simulink model "part4_Final_Project"  (R2016b)
settings: Solver=FixedStepDiscrete  StartTime=0.0  StopTime=inf  FixedStep=.03  RelTol=1e-3  EnableMultiTasking=on
undefined symbols (not defined in the file or in its folder): Klqr
libraries: arduinolib x2, simulink x1
settings Model: SimulationMode=external  ExtModeTrigDuration=2  Creator=008528533  LastModifiedBy=Mac
settings DataIOCC: LimitDataPoints=on  SaveFormat=Array
settings OptimizationCC: LifeSpan=1
settings DebuggingCC: UnderspecifiedInitializationDetection=Classic  MergeDetectMultiDrivingBlocksExec=none  SFUnexpectedBacktrackingDiag=warning  SFNoUnconditionalDefaultTransitionDiag=warning  SFExecutionAtInitializationDiag=none
settings HardwareCC: ProdBitPerInt=16  ProdBitPerPointer=8  ProdBitPerSizeT=16  ProdBitPerPtrDiffT=16  ProdLargestAtomicFloat=None  ProdWordSize=8  ProdHWDeviceType=Atmel->AVR
settings ModelReferenceCC: PropagateSignalLabelsOutOfModel=off
settings RTWCC: SystemTargetFile=realtime.tlc  GenerateMakefile=off  TemplateMakefile=realtime.tmf  Description=Run on Target Hardware  RTWVerbose=off
settings STFCustomTargetCC: TargetLibSuffix=.a  GenerateSampleERTMain=on  ERTCustomFileBanners=on  SupportNonInlinedSFcns=off  RemoveResetFunc=on  SupportVariableSizeSignals=on  MATLABClassNameForMDSCustomization=Simulink.SoftwareTarget.ERTCustomization  GRTInterface=off  SystemTargetFile=realtime.tlc
settings ERTTargetCC: GenerateSampleERTMain=on  ParMdlRefBuildCompliant=off  CompOptLevelCompliant=off  ConcurrentExecutionCompliant=off  CombineOutputUpdateFcns=off  ERTFirstTimeCompliant=off  SupportContinuousTime=on  SupportVariableSizeSignals=on  ModelStepFunctionPrototypeControlCompliant=off  CPPClassGenCompliant=off  UseToolchainInfoCompliant=off  ExtMode=on  ExtModeTransport=3  ExtModeMexFile=ext_serial_win32_comm_rtt  ExtModeMexArgs=0 8 115200 30  ERTSrcFileBannerTemplate=realtime_code_template.cgt  ERTHdrFileBannerTemplate=realtime_code_template.cgt  ERTDataSrcFileTemplate=realtime_code_template.cgt  ERTDataHdrFileTemplate=realtime_code_template.cgt  ERTCustomFileTemplate=realtime_file_process.tlc  ConvertIfToSwitch=off  SuppressUnreachableDefaultCases=off
settings ConfigComp: CovMetricSettings=dw  CovHtmlReporting=on  CovSaveCumulativeToWorkspaceVar=on  CovSaveSingleToWorkspaceVar=on  CovExternalEMLEnable=off

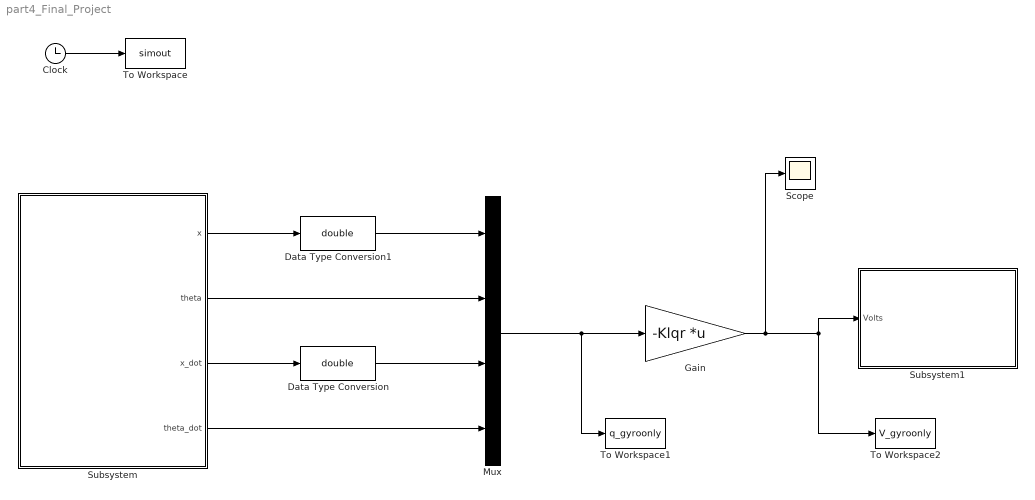
== system part4_Final_Project ==
  Clock : Clock
  Data Type Conversion : DataTypeConversion  OutDataTypeStr=double
  Data Type Conversion1 : DataTypeConversion  OutDataTypeStr=double
  Gain : Gain  Gain=-Klqr  Multiplication=Matrix(K*u)
  Mux : Mux
  Scope : Scope
  Subsystem : Subsystem
  Subsystem1 : Subsystem
  To Workspace : ToWorkspace  VariableName=simout  SaveFormat=Timeseries  SampleTime=-1
  To Workspace1 : ToWorkspace  VariableName=q_gyroonly  SampleTime=-1
  To Workspace2 : ToWorkspace  VariableName=V_gyroonly  SampleTime=-1
  wires:
  Clock/1 -> To Workspace/1
  Subsystem/1(x) -> Data Type Conversion1/1
  Data Type Conversion1/1 -> Mux/1
  Subsystem/2("theta ") -> Mux/2
  Subsystem/3(x_dot) -> Data Type Conversion/1
  Data Type Conversion/1 -> Mux/3
  Subsystem/4("theta_dot ") -> Mux/4
  Mux/1 -> To Workspace1/1, Gain/1
  Gain/1 -> Scope/1, To Workspace2/1, Subsystem1/1(Volts)

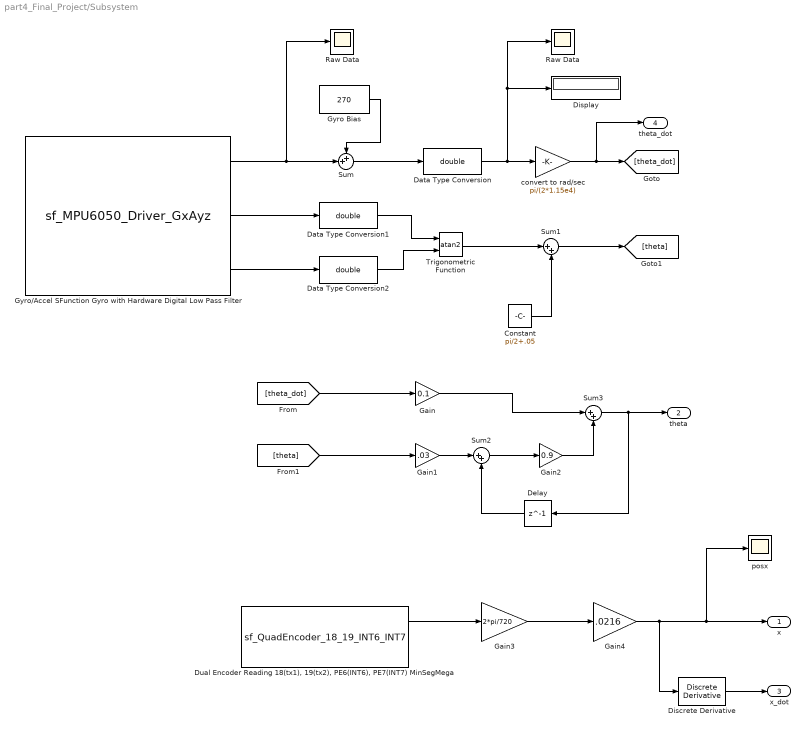
== system part4_Final_Project/Subsystem ==
  Constant : Constant  Value=pi/2+.05
  Data Type Conversion : DataTypeConversion  OutDataTypeStr=double
  Data Type Conversion1 : DataTypeConversion  OutDataTypeStr=double
  Data Type Conversion2 : DataTypeConversion  OutDataTypeStr=double
  Delay : Delay  DelayLength=1
  Discrete Derivative : simulink/Discrete/Discrete Derivative  gainval=1.0  ICPrevScaledInput=0.0  InputProcessing=Inherited  OutMin=[]  OutMax=[]  OutDataType=fixdt(1, 16)  OutScaling=2^-10  DoSatur=off
  Display : Display
  "Dual Encoder Reading 18(tx1), 19(tx2), PE6(INT6), PE7(INT7) MinSegMega " : S-Function  InitFcn=try, set_param(gcb,'FunctionName','sf_QuadEncoder_18_19_INT6_INT7'), end  FunctionName=sf_QuadEncoder_18_19_INT6_INT7  Parameters=uint8([0 1]),uint8([18 6]),uint8([19 7])  SFunctionModules=sf_QuadEncoder_18_19_INT6_INT7_wrapper  SFunctionDeploymentMode=off  EnableBusSupport=off  mask(S-Function Builder){}
      mask init:
      | val = [[.9  0.75 0.75 1 1 .9 .9 1]',[1 1 0.75 0.75 .9 .9 1 .9]'];try , sys = get_param(gcb,'SfunBuilderFcnName');if isempty(sys), sys = get_param(gcb,'FunctionName'); end,catch, sys = get_param(gcb,'FunctionName'); end
      settings: CopyFcn=set_param(gcbh,'LinkStatus','none')  PreSaveFcn=try, set_param(gcb,'FunctionName','sf_QuadEncoder_18_19_INT6_INT7'), end  OpenFcn=sfunctionwizard(gcbh)
      mask Display: plot(val(:,1),val(:,2)),disp(sys), port_label('output',1,'pos1'), port_label('output',2,'pos2')
  Gain : Gain  Gain=0.1
  Gain1 : Gain  Gain=.03
  Gain2 : Gain  Gain=0.9
  Gain3 : Gain  Gain=2*pi/720
  Gain4 : Gain  Gain=.0216
  Gyro Bias : Constant  Value=270
  Gyro/Accel SFunction Gyro with Hardware Digital Low Pass Filter : S-Function  InitFcn=try, set_param(gcb,'FunctionName','sf_MPU6050_Driver_GxAyz'), end  FunctionName=sf_MPU6050_Driver_GxAyz  SFunctionModules=sf_MPU6050_Driver_GxAyz_wrapper  SFunctionDeploymentMode=off  EnableBusSupport=off  mask(S-Function Builder){}
      mask help: Simulink:masks:SFunctionBuilder_MD
      mask init: same as part4_Final_Project/Subsystem/Dual Encoder Reading 18(tx1), 19(tx2), PE6(INT6), PE7(INT7) MinSegMega 
      settings: CopyFcn=set_param(gcbh,'LinkStatus','none')  PreSaveFcn=try, set_param(gcb,'FunctionName','sf_MPU6050_Driver_GxAyz'), end  OpenFcn=sfunctionwizard(gcbh)
      mask Display: plot(val(:,1),val(:,2)),disp(sys), port_label('output',1,'x_vel'), port_label('output',2,'y_acc'), port_label('output',3,'z_acc')
  Raw Data : Scope
  "Raw Data " : Scope
  Sum : Sum  Inputs=++|
  Sum1 : Sum  Inputs=|++
  Sum2 : Sum  Inputs=|++
  Sum3 : Sum  Inputs=|++
  Trigonometric Function : Trigonometry  Operator=atan2
  convert to rad/sec : Gain  Gain=pi/(2*1.15e4)
  posx : Scope
  x : Outport
  "theta " : Outport  Port=2
  x_dot : Outport  Port=3
  "theta_dot " : Outport  Port=4
  wires:
  Gyro Bias/1 -> Sum/1
  Sum/1 -> Data Type Conversion/1
  Data Type Conversion/1 -> Raw Data/1, Display/1, convert to rad/sec/1
  convert to rad/sec/1 -> "theta_dot "/1, [theta_dot]
  Gyro/Accel SFunction Gyro with Hardware Digital Low Pass Filter/1 -> "Raw Data "/1, Sum/2
  Gyro/Accel SFunction Gyro with Hardware Digital Low Pass Filter/3 -> Data Type Conversion2/1
  Gyro/Accel SFunction Gyro with Hardware Digital Low Pass Filter/2 -> Data Type Conversion1/1
  Data Type Conversion1/1 -> Trigonometric Function/1
  Trigonometric Function/1 -> Sum1/1
  Data Type Conversion2/1 -> Trigonometric Function/2
  [theta_dot] -> Gain/1
  Constant/1 -> Sum1/2
  Sum1/1 -> [theta]
  [theta] -> Gain1/1
  Sum3/1 -> "theta "/1, Delay/1
  Delay/1 -> Sum2/2
  Sum2/1 -> Gain2/1
  Gain1/1 -> Sum2/1
  Gain/1 -> Sum3/1
  Gain2/1 -> Sum3/2
  Gain3/1 -> Gain4/1
  "Dual Encoder Reading 18(tx1), 19(tx2), PE6(INT6), PE7(INT7) MinSegMega "/1 -> Gain3/1
  Gain4/1 -> posx/1, x/1, Discrete Derivative/1
  Discrete Derivative/1 -> x_dot/1

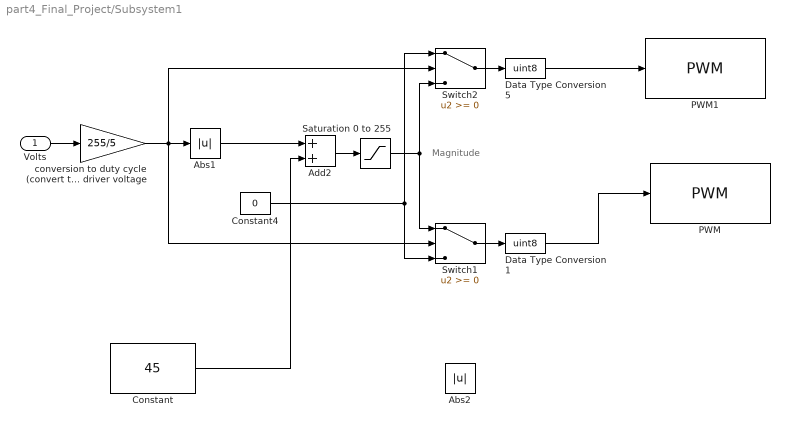
== system part4_Final_Project/Subsystem1 ==
  note: Magnitude
  Volts : Inport
  Abs1 : Abs
  Abs2 : Abs
  Add2 : Sum
  Constant : Constant  Value=45
  Constant4 : Constant  Value=0
  Data Type Conversion1 : DataTypeConversion  OutDataTypeStr=uint8
  Data Type Conversion5 : DataTypeConversion  OutDataTypeStr=uint8
  PWM : arduinolib/PWM  pinNumber=45  blockPlatform=arduino
  PWM1 : arduinolib/PWM  pinNumber=44  blockPlatform=arduino
  Saturation 0 to 255 : Saturate  UpperLimit=255  LowerLimit=0
  Switch1 : Switch
  Switch2 : Switch
  conversion to duty cycle (convert to int) denominator is motor driver voltage : Gain  Gain=255/5  OutDataTypeStr=int16
  wires:
  Volts/1 -> conversion to duty cycle (convert to int) denominator is motor driver voltage/1
  conversion to duty cycle (convert to int) denominator is motor driver voltage/1 -> Abs1/1, Switch2/2, Switch1/2
  Switch2/1 -> Data Type Conversion5/1
  Constant4/1 -> Switch1/3, Switch2/1
  Switch1/1 -> Data Type Conversion1/1
  Data Type Conversion1/1 -> PWM/1
  Data Type Conversion5/1 -> PWM1/1
  Constant/1 -> Add2/2
  Add2/1 -> Saturation 0 to 255/1
  Abs1/1 -> Add2/1
  Saturation 0 to 255/1 -> Switch2/3, Switch1/1
